simulink model "Simulacion_stepper"  (R2025b)
settings: Solver=ode4  StartTime=0.0  StopTime=Time_simulation  FixedStep=1/frecuency_simulation  RelTol=1e-3
InitFcn:
  | %%InitFcn();
StopFcn:
  | %%FinishFcn
model workspace (MAT data in the model file):
  Ts_stepper = 0.001
values from neighbouring files (symbols this model uses):
  B = motor_params.B_internal    [bode.m]    (also in current_observer.m = 0.0005; discretizacion.m = [ 1/L, 0; ekf_4_estados.m = params.B; obs_ctrl_back_emf_ext.m = [1/L 0)
  frecuency_simulation = 10e3    (= 10000)    [InitFcn.m]
  J = motor_params.J_internal    [bode.m]    (also in current_observer.m = 0.008; ekf_4_estados.m = params.J; obs_ctrl_back_emf_ext.m = 0.008; obs_y_contrl_back_emd.m = 0.008)
  Ke = 0.0055    [current_observer.m]    (also in ekf_4_estados.m = params.Ke; observer.m = Pvec(3); salient_motor.m = 0.0066)
  Ki_d = PI_dq_params.Ki_d_salient    [bode.m]
  Ki_q = PI_dq_params.Ki_q_salient    [bode.m]
  Ki_w = (wn_w^2)*J_var/Kt    [Barrido_B.m]    (also in Barrido_J.m; bode.m = PI_MTPA_params.Ki_w)
  Kp_d = PI_dq_params.Kp_d_salient    [bode.m]
  Kp_q = PI_dq_params.Kp_q_salient    [bode.m]
  Kp_w = (2*shi_w*wn_w*J_var)/Kt    [Barrido_B.m]    (also in Barrido_J.m; bode.m = PI_MTPA_params.Kp_w)
  Kt = Nr*Ke    (= 0.275)    [current_observer.m]    (also in ekf_4_estados.m = params.Kt; frecuencia_max.m = 0.33; observer.m = Pvec(4); salient_motor.m = 0.33)
  L = place(A', C', 10*eig(A)).'    [current_observer.m]    (also in desfase.m = lags(k); discretizacion.m = 0.01; frecuencia_max.m = 0.006; obs_ctrl_back_emf_ext.m = 0.006)
  P = motor_params.P    [bode.m]    (also in ekf_4_estados.m = P_pred; frecuencia_max.m = 50; salient_motor.m = 50)
  R = motor_params.R    [bode.m]    (also in current_observer.m = 3.4; discretizacion.m = 3.4; ekf_4_estados.m = params.R; frecuencia_max.m = 3.4)
  sample_time = 1/frecuency_simulation    (= 0.0001)    [InitFcn.m]
  Ts_current = 1/f_current    (= 0.0001)    [InitFcn.m]
  Ts_Wm = Ts_current*10    (= 0.001)    [InitFcn.m]
  Vdc = 24    [InitFcn.m]    (also in frecuencia_max.m = 12)
undefined symbols (not defined in the file or in its folder): DiscIntNeverNeededParam, EKF_params, motor_params, RI_base
libraries: simulink x8, mcbeeMathTransformLib x3, spspowerguiLib x1
(part 4 of 5)

== matlab function Simulacion_stepper/Triggered Subsystem2/MATLAB Function ==
  data: U input; x_out output; X input; Ts input; Ke input; Kt input; R input; J input; Ld input; Lq input; Nr input; B input; wh input; b0 input; b1 input; b2 input; a1 input; a2 input; HFI_flag input
function x_out = ekf_dq_5states_tightly_coupled( ...
    U, X, Ts, Ke, Kt, R, J, Ld, Lq, Nr, B, ...
    wh, b0, b1, b2, a1, a2, HFI_flag)

% =========================================================================
% EKF 5 ESTADOS TIGHTLY COUPLED CON HFI
%
% Estados:
%
%   x = [Id; Iq; Wm; theta_e; Tx]
%
% theta_e:
%   Ángulo eléctrico.
%
% Mediciones:
%
%   y_med  = [Ia; Ib; 0]
%   y_pred = [Ia_pred; Ib_pred; eps_norm]
%
% La tercera medición impone:
%
%   eps_norm -> 0
%
% IMPORTANTE:
%   Para que esta formulación sea físicamente coherente, eps_norm debe
%   representar aproximadamente un error angular eléctrico.
% =========================================================================

% Parámetros no utilizados actualmente:
% N_steps, Tdtm, beta0, beta1, beta2

Ts_eff = max(Ts, 1e-9);

% =========================================================================
% ESTADOS PERSISTENTES
% =========================================================================

persistent x_hat
persistent P
persistent Qk

persistent xa1 xa2 ya1 ya2
persistent xb1 xb2 yb1 yb2

persistent t_h
persistent eps_f

if isempty(x_hat)

    % Estado inicial
    x_hat = zeros(5,1);

    % Covarianza inicial
    P = diag([ ...
        1e-6, ...   % Id
        1e-6, ...   % Iq
        1e-6, ...   % Wm
        1e-9, ...   % theta_e
        1e-5]);     % Tx

    % Ruido del proceso
    Qk = diag([ ...
        1e-8, ...   % Id
        1e-8, ...   % Iq
        1e-8, ...   % Wm
        1e-12, ...   % theta_e
        1e-5]);     % Tx

    % Estados del BPF de Ia
    xa1 = 0;
    xa2 = 0;
    ya1 = 0;
    ya2 = 0;

    % Estados del BPF de Ib
    xb1 = 0;
    xb2 = 0;
    yb1 = 0;
    yb2 = 0;

    % Estados HFI
    t_h   = 0;
    eps_f = 0;

end

% =========================================================================
% 1. MEDICIONES Y ENTRADAS
% =========================================================================

Ia_raw = X(1);
Ib_raw = X(2);

Va = U(1);
Vb = U(2);

% =========================================================================
% 2. ESTADOS ACTUALES
% =========================================================================

Id = x_hat(1);
Iq = x_hat(2);
Wm = x_hat(3);

% El estado angular se conserva continuo internamente
theta_e_state = x_hat(4);

Tx = x_hat(5);

% Ángulo envuelto únicamente para trigonometría
theta_e = wrap_pi(theta_e_state);

c = cos(theta_e);
s = sin(theta_e);

% =========================================================================
% 3. TRANSFORMACIÓN DE TENSIONES AL MARCO dq
% =========================================================================

Vd =  Va*c + Vb*s;
Vq = -Va*s + Vb*c;

% =========================================================================
% 4. PREDICCIÓN DEL ESTADO
% =========================================================================

We = Nr*Wm;

dId = ( ...
      Vd ...
    - R*Id ...
    + We*Lq*Iq) / Ld;

dIq = ( ...
      Vq ...
    - R*Iq ...
    - We*Ld*Id ...
    - Ke*Wm) / Lq;

% Torque electromagnético
Te = Kt*Iq + Nr*(Lq-Ld)*Id*Iq;

% Tx representa la carga desconocida
dWm = (Te - B*Wm - Tx)/J;

% Alternativa si Tdtm es una carga conocida:
%
% dWm = (Te - B*Wm - Tdtm - Tx)/J;

x_pred = zeros(5,1);

x_pred(1) = Id + Ts_eff*dId;
x_pred(2) = Iq + Ts_eff*dIq;
x_pred(3) = Wm + Ts_eff*dWm;

% Ángulo eléctrico continuo
x_pred(4) = theta_e_state + Ts_eff*Nr*Wm;

% Torque desconocido como random walk
x_pred(5) = Tx;

% =========================================================================
% 5. JACOBIANA DE TRANSICIÓN
% =========================================================================

A = [ ...
    -R/Ld, ...
     Nr*Wm*Lq/Ld, ...
     Nr*Lq*Iq/Ld, ...
     Vq/Ld, ...
     0;

    -Nr*Wm*Ld/Lq, ...
    -R/Lq, ...
    -(Nr*Ld*Id + Ke)/Lq, ...
    -Vd/Lq, ...
     0;

     Nr*(Lq-Ld)*Iq/J, ...
     (Kt + Nr*(Lq-Ld)*Id)/J, ...
    -B/J, ...
     0, ...
    -1/J;

     0, ...
     0, ...
     Nr, ...
     0, ...
     0;

     0, ...
     0, ...
     0, ...
     0, ...
     0];

Phi = eye(5) + Ts_eff*A;

P_pred = Phi*P*Phi' + Qk;
P_pred = 0.5*(P_pred + P_pred');

% =========================================================================
% 6. FILTRO PASABANDA DE LAS CORRIENTES HFI
% =========================================================================

Iah = ...
      b0*Ia_raw ...
    + b1*xa1 ...
    + b2*xa2 ...
    - a1*ya1 ...
    - a2*ya2;

xa2 = xa1;
xa1 = Ia_raw;

ya2 = ya1;
ya1 = Iah;

Ibh = ...
      b0*Ib_raw ...
    + b1*xb1 ...
    + b2*xb2 ...
    - a1*yb1 ...
    - a2*yb2;

xb2 = xb1;
xb1 = Ib_raw;

yb2 = yb1;
yb1 = Ibh;

% =========================================================================
% 7. PROYECCIÓN HFI RESPECTO DEL ÁNGULO PREDICHO
% =========================================================================

theta_e_pred = wrap_pi(x_pred(4));

ch = cos(theta_e_pred);
sh = sin(theta_e_pred);

% Componente HFI sobre el eje q estimado
Iqh = -Iah*sh + Ibh*ch;

% =========================================================================
% 8. DEMODULACIÓN SÍNCRONA
% =========================================================================

if wh > 0

    t_h = t_h + Ts_eff;

    T_hfi = 2*pi/wh;

    if t_h >= T_hfi
        t_h = t_h - T_hfi*floor(t_h/T_hfi);
    end

    % Verificar signo y fase según la señal efectivamente inyectada
    eps_raw = -Iqh*cos(wh*t_h);

else

    t_h = 0;
    eps_raw = 0;

end

% =========================================================================
% 9. FILTRO PASABAJOS DEL ERROR HFI
% =========================================================================

f_lpf_hfi = 50;

tau_lpf   = 1/(2*pi*f_lpf_hfi);
alpha_lpf = Ts_eff/(Ts_eff + tau_lpf);

eps_f = eps_f + alpha_lpf*(eps_raw - eps_f);

% =========================================================================
% 10. NORMALIZACIÓN DEL ERROR HFI
% =========================================================================

DeltaL = Lq - Ld;
Lavg   = 0.5*(Ld + Lq);

if abs(DeltaL) < 1e-12 || Lavg <= 0

    eps_norm = 0;

else

    saliency = DeltaL/Lavg;

    % Formulación original:
    %
    % Se supone empíricamente que eps_norm aproxima un error angular.
    %
    % Atención: dividir por la saliencia no garantiza que el resultado
    % tenga unidades de radianes.
    % Formulación original:
    eps_norm = eps_f/abs(saliency);
    
    % NUEVO: Límite estricto de seguridad para evitar retroalimentación positiva
    max_eps = pi/4; % 45 grados eléctricos
    eps_norm = max(-max_eps, min(max_eps, eps_norm));

end

if ~HFI_flag
    eps_norm = 0;
end

% Protección numérica
if ~isfinite(eps_norm)
    eps_norm = 0;
end

% =========================================================================
% 11. PREDICCIÓN DE LAS MEDICIONES DE CORRIENTE
% =========================================================================

Id_p = x_pred(1);
Iq_p = x_pred(2);

cp = cos(theta_e_pred);
sp = sin(theta_e_pred);

Ia_pred = Id_p*cp - Iq_p*sp;
Ib_pred = Id_p*sp + Iq_p*cp;

% =========================================================================
% 12. VECTOR DE MEDICIÓN DE TRES COMPONENTES
% =========================================================================
%
% La tercera medición impone que el error HFI sea cero.
% =========================================================================

y_med = [ ...
    Ia_raw;
    Ib_raw;
    0];

y_pred = [ ...
    Ia_pred;
    Ib_pred;
    eps_norm];

innov = y_med - y_pred;

% Equivalente:
%
% innov(1) = Ia_raw - Ia_pred
% innov(2) = Ib_raw - Ib_pred
% innov(3) = -eps_norm

% =========================================================================
% 13. JACOBIANA DE MEDICIÓN
% =========================================================================

dIa_dtheta_e = -Id_p*sp - Iq_p*cp;
dIb_dtheta_e =  Id_p*cp - Iq_p*sp;

% Si:
%
% eps_norm ≈ theta_real - theta_estimado
%
% entonces:
%
% d(eps_norm)/d(theta_estimado) ≈ -1
dEps_dtheta_e = -1;

Ck = [ ...
    cp, -sp, 0, dIa_dtheta_e, 0;
    sp,  cp, 0, dIb_dtheta_e, 0;
    0,   0,  0, dEps_dtheta_e, 0];

% =========================================================================
% 14. COVARIANZA DE LAS TRES MEDICIONES
% =========================================================================

sigma_Ia = 0.1;
sigma_Ib = 0.1;

if HFI_flag

    sigma_HFI = 0.25;

else

    % El HFI queda prácticamente ignorado
    sigma_HFI = 1e6;

end

Rk = diag([ ...
    sigma_Ia^2, ...
    sigma_Ib^2, ...
    sigma_HFI^2]);

% =========================================================================
% 15. GANANCIA DE KALMAN
% =========================================================================

Sk = Ck*P_pred*Ck' + Rk;
Sk = 0.5*(Sk + Sk');

% Evitar inversión explícita
Lk = (P_pred*Ck')/Sk;

% =========================================================================
% 16. CORRECCIÓN TIGHTLY COUPLED
% =========================================================================

x_corr_ekf = x_pred + Lk*innov;

% No se envuelve internamente para mantener continuidad angular
% x_corr_ekf(4) permanece continuo.

% =========================================================================
% 17. ACTUALIZACIÓN DE COVARIANZA: FORMA DE JOSEPH
% =========================================================================

I5 = eye(5);

P = ...
    (I5 - Lk*Ck)*P_pred*(I5 - Lk*Ck)' ...
    + Lk*Rk*Lk';

P = 0.5*(P + P');

% =========================================================================
% 18. PROTECCIÓN NUMÉRICA
% =========================================================================

if any(~isfinite(x_corr_ekf)) || any(~isfinite(P(:)))

    x_corr_ekf = x_pred;
    P = P_pred;

end

% =========================================================================
% 19. ACTUALIZACIÓN DEL ESTADO
% =========================================================================

x_hat = x_corr_ekf;

% =========================================================================
% 20. SALIDA
% =========================================================================

x_out = x_hat;

% Solo la salida angular se envuelve
x_out(4) = wrap_pi(x_hat(4));

end

% =========================================================================
% FUNCIÓN AUXILIAR
% =========================================================================

function out = wrap_pi(in)

out = atan2(sin(in), cos(in));

end

== matlab function Simulacion_stepper/Triggered Subsystem2/MATLAB Function1 ==
  data: U input; x_corr output; X input; Ts input; Kt input; R input; J input; L input; Nr input; B input; Ke input
function x_corr = ekf_5var(U,X,Ts,Kt,R,J,L,Nr,B,Ke)
persistent x_hat P x_pred
%%  x_hat son los estados predichos
%%  x_corr es la salida corregida
%%  P_pre ó Sum_less es la covarianza predicha
%%  P ó sum_more es la covarianza
%%  Rk ó sum_v es la covarianza de incertidumbre del sensor




 %%Iniciamos calculando X_hat[k-1]
 if isempty(x_hat)
     x_hat = zeros(5,1);
     P = diag([1e-4 1e-4 1e-6 1e-10 1e-4]);
     x_corr = zeros(5,1);
     x_pred = zeros(5,1);


 end

Qk = diag([1e-4 1e-4 1e-4 1e-10 1e-6]);
Rk = diag([5e-4 5e-4]);   % ruido de medición

%%1A
%%Predicción
Ia = x_hat(1);
Ib = x_hat(2);
Wm = x_hat(3);
Th_m = x_hat(4);
Tx = x_hat(5);

Th_e = Nr*Th_m;
S = sin(Th_e);
C = cos(Th_e);

Va = U(1);
Vb = U(2);

dx = zeros(5,1);
dx(1) = (Va - R*Ia + Ke*Wm*S)/L;
dx(2) = (Vb - R*Ib - Ke*Wm*C)/L;
dx(3) = (Kt*(Ib*C-Ia*S) -Tx)/J;
dx(4) = Wm;
dx(5) = 0;
x_pred = x_hat + Ts*dx;
x_pred(4) = wrap_2pi(x_pred(4));

%%Calculamos el jacobiano
RL = R/L;
uno = Ke*S;
dos = Ke*C;

A = [-RL 0   (uno/L) (dos*Nr*Wm/L) 0;
 0  -RL   -dos/L    uno*Nr*Wm/L  0;
 -uno/J dos/J -1/J -Kt*Nr*(Ia*C+Ib*S)/J -1/J;
 0 0 1 0 0;
 0 0 0 0 0];

A_hat = eye(5) + Ts*A;
A_hat_T = transpose(A_hat);

%%1B COVARIANZA PREDICHA
P_pred = A_hat * P * A_hat_T + Qk; 


%%1C PREDECIMOS LA SALIDA DEL SISTEMA
Ck = [1 0 0 0 0;
      0 1 0 0 0];
Ck_T = transpose(Ck);
y_pred = Ck*x_pred;

%%2A calculamos la matriz Lk
%%Lk = P_pred *Ck_T * inv(Ck*P_pred*Ck_T + sum_v)
Sk = Ck*P_pred*Ck_T + Rk;
Lk = P_pred * Ck_T /Sk;

%%2B Actualizamos los estados estados corregidos en función de L


y_meas = [X(1);X(2)];

innov = y_meas - y_pred;
x_corr = x_pred + Lk*(innov);
x_corr(4) = wrap_2pi(x_corr(4));
%%actualizamos la covarianza y guardamos el estado
x_hat = x_corr;
Lk_T = transpose(Lk);
P = P_pred - Lk*Sk*Lk_T;
P_T = transpose(P);
P = 0.5 * (P + P_T);

== matlab function Simulacion_stepper/Triggered Subsystem2/MATLAB Function2 ==
  data: U input size=2; x_corr output; Y input size=2; Ts input; Kt input; R input; J input; L input; Nr input; B input
function x_corr = SPKF_4var(U,Y,Ts,Kt,R,J,L,Nr,B)
persistent x_hat P  alpham alphac Qk Rk h
%%  x_hat son los estados predichos
%%  x_corr es la salida corregida
%%  P_pre ó Sum_less es la covarianza predicha
%%  P ó sum_more es la covarianza
%%  Rk ó sum_v es la covarianza de incertidumbre del sensor


Nx = 4; %%Números de estados
Nw = 4; %% Incertidumbres de estado
Ny = 2; %% Incertidumbre de mediciones
Na = Nx+Nw+Ny;


%%Los métodos de sigma-point pueden diferir al utilizar las variables
%%alpha. Existen 2 métodos:

%% Método |    Sigma       |     alpha_m_0      | alpha_m_k         |           alpha_c_0               | alpha_c_k |
%% UKF    | sqrt(L+lambda) |  lambda/(L+Lambda) | 1/(2*(L+Lambda))  | alpha_m_0 + (1-alpha^2 + betha)   | alpha_m_k |
%% CDKF   |    h           |   (h^2 - L)/h^2    |  1/(2*h^2)        | alpha_m_0                         | alpha_m_k |
 %%Iniciamos calculando X_hat[k-1]
 if isempty(x_hat)
    
     %%Utilizamos el CDKF, con h = sqrt(Nxa); 
        x_hat = zeros(Nx,1);
        h =sqrt(Na);
        alpham = ones(2*Na+1,1) * (1/(2*h^2));
        alpham(1) = (h^2 - Na)/(h^2);   % peso del sigma central
        alphac = alpham;             
     %%Valores de covarianza
     P = diag([1e-2 1e-2 1e-6 1e-12 ]);
     Qk = diag([1e-2 1e-2 1e-8 1e-12 ]);
     Rk = [1e-4 0; 0 1e-4];
 end
    
     x_corr = zeros(Nx,1);
     x_pred = zeros(Nx,1);
     x_hat_a = zeros(Na,1);
     X_minus = zeros(Nx,2*Na+1);
     Y_minus = zeros(Ny,2*Na+1);
%%Ciclo de 2*Na+1
%%Aun que deberiamos hacer un ciclo for, en matlab se hace solo asi que no
%%es necesario

%% 1A-I Creamos el vector de estados extendidos
x_hat_a = [x_hat;zeros(Nw,1);zeros(Ny,1)]; 


%% 1A-II Conseguimos el factor de cholesky


%%Creamos la matriz de covarianza extendidas, el cual es de la forma
%%             [P   0    0]
%%     P_a =   [0   Qk   0]
%%             [0   0   Rk]

P_a = blkdiag(P,Qk,Rk);
Sa = chol(P_a,"lower");

%% 1A-III generamos los sigma points
%% Queda de la forma [x_hat_a, x_hat_a + h*S,x_hat_a - h*S] (Por eso es 2*Nxa+1 = N)
%% Al usar x_a x_a(:,ones(1,Na)) creamos una matriz de la forma [x_a,x_a...x_a], que es de tamaño (Na)x(2*Na+1)
%% Posteriormente, se le suma un vector de [0,+h*S,-h*S]
%% Cómo S es del tamaño (Nxa)x(Nxa), el total es de (2*Na+1 = N)
X =  x_hat_a(:,ones(1,2*Na+1)) + h*[zeros(Na,1), Sa, -Sa];

%% 1A-IV Calculamos las ecuaciones de estado
Va = U(1);
Vb = U(2);


for k=1:2*Na+1

  % --- separar estado, ruido de proceso y ruido de medición ---


xk = X(1:Nx,k);                     % [Ia; Ib; Wm; Th_m]
wk = X(Nx+1 : Nx+Nw,k);             % ruido de proceso (4x1)
vk = X(Nx+Nw+1 : end,k);            % ruido de medición (2x1)    

Ia = xk(1);
Ib = xk(2);
Wm = xk(3);
Th_m = xk(4);

Th_e = Nr*Th_m;
S = sin(Th_e);
C = cos(Th_e);


dx1 = (Va - R*Ia + Kt*Wm*S)/L;
dx2 = (Vb - R*Ib - Kt*Wm*C)/L;
dx3 = (Kt*(Ib*C-Ia*S)-B*Wm)/J;
dx4 = Wm;

%Calculamos el paso siguiente mediante euler
%% X_minus corresponde a la matriz que contiene todos los sigma-points distribuidos en los estados del sistema no-extendido (Nx)x(Na)
X_minus(1,k) = Ia + Ts*dx1+ wk(1);
X_minus(2,k) = Ib + Ts*dx2 + wk(2);
X_minus(3,k) = Wm + Ts*dx3 + wk(3);
X_minus(4,k) = Th_m + Ts*dx4 + wk(4);
%%X_minus(4,k) = wrap_2pi(X_minus(4,k));

Y_minus(1,k) = X_minus(1,k) + vk(1);
Y_minus(2,k) = X_minus(2,k) + vk(2);

end
%% 1B Reconstrucción de la media
%% Esta matriz contiene la media de todos los estados. (Nx)x(1)
x_pred = X_minus*alpham;
y_pred = Y_minus*alpham;
%%  Reconstrucción de la covarianza

%% Acá lo que hacemos es copiar la media N veces, para poder realizar la resta.
%%Pero realmente debería ser un for de [Xs(i,k)= X_minus(i,k) - x_pred(i)],
%%dónde K es cada variable de estado (Nx)
%% Xs es una matriz de desviación respecto a la media. Es necesario para construir la covarianza P
Xs = X_minus - x_pred(:,ones([1 2*Na+1])); 
Ys = Y_minus - y_pred(:,ones([1 2*Na+1]));

Xs_T = transpose(Xs);
Ys_T = transpose(Ys);
%%Calculamos la matriz de covarianza, pero hay que considerar que como
%%diag(alphac) es una matriz llena de diagonales, uno puede reducir la
%%cantidad de cómputo.
P_pred = Xs*diag(alphac)*Xs_T;
Pyy = Ys* diag(alphac)* Ys_T;
Pxy = Xs*diag(alphac)*Ys_T;
Lk = Pxy/Pyy;
Lk_T = transpose(Lk);
%% 2B Leemos la medición y actualizamos
x_corr = x_pred + Lk*(Y - y_pred);
x_corr(4) = wrap_2pi(x_corr(4));
%%Guardamos los valores de x_hat para mantenerlos
x_hat = x_corr; 
%% 2C Actualizamos la covarianza
P = P_pred - Lk*Pyy*Lk_T;
P_T = transpose(P);
P = 0.5 * (P + P_T);

== matlab function Simulacion_stepper/Triggered Subsystem2/MATLAB Function3 ==
  data: U input size=2; x_corr output; Y input size=2; Ts input; Kt input; R input; J input; L input; Nr input; B input
function x_corr = SPKF_5var(U,Y,Ts,Kt,R,J,L,Nr,B)
persistent x_hat P x_pred alpham alphac Qk Rk h
%%  x_hat son los estados predichos
%%  x_corr es la salida corregida
%%  P_pre ó Sum_less es la covarianza predicha
%%  P ó sum_more es la covarianza
%%  Rk ó sum_v es la covarianza de incertidumbre del sensor


Nx = 5; %%Números de estados
Nw = 5; %% Incertidumbres de estado
Ny = 2; %% Incertidumbre de mediciones
Na = Nx+Nw+Ny;


%%Los métodos de sigma-point pueden diferir al utilizar las variables
%%alpha. Existen 2 métodos:

%% Método |    Sigma       |     alpha_m_0      | alpha_m_k         |           alpha_c_0               | alpha_c_k |
%% UKF    | sqrt(L+lambda) |  lambda/(L+Lambda) | 1/(2*(L+Lambda))  | alpha_m_0 + (1-alpha^2 + betha)   | alpha_m_k |
%% CDKF   |    h           |   (h^2 - L)/h^2    |  1/(2*h^2)        | alpha_m_0                         | alpha_m_k |
 %%Iniciamos calculando X_hat[k-1]
 if isempty(x_hat)
    
     %%Utilizamos el CDKF, con h = sqrt(Nxa); 
        x_hat = zeros(Nx,1);
        h =sqrt(Na);
        alpham = ones(2*Na+1,1) * (1/(2*h^2));
        alpham(1) = (h^2 - Na)/(h^2);   % peso del sigma central
        alphac = alpham;             
     %%Valores de covarianza
     P = diag([1e-2 1e-2 1e-4 1e-8 1e-12]);
     Qk = diag([1e-2 1e-2 1e-6 1e-8 1e-12]);
     Rk = [1e-4 0; 0 1e-4];
 end
    
     x_corr = zeros(Nx,1);
     x_pred = zeros(Nx,1);
     x_hat_a = zeros(Na,1);
     X_minus = zeros(Nx,2*Na+1);
     Y_minus = zeros(Ny,2*Na+1);
%%Ciclo de 2*Na+1
%%Aun que deberiamos hacer un ciclo for, en matlab se hace solo asi que no
%%es necesario

%% 1A-I Creamos el vector de estados extendidos
x_hat_a = [x_hat;zeros(Nw,1);zeros(Ny,1)]; 


%% 1A-II Conseguimos el factor de cholesky


%%Creamos la matriz de covarianza extendidas, el cual es de la forma
%%             [P   0    0]
%%     P_a =   [0   Qk   0]
%%             [0   0   Rk]

P_a = blkdiag(P,Qk,Rk);
Sa = chol(P_a,"lower");

%% 1A-III generamos los sigma points
%% Queda de la forma [x_hat_a, x_hat_a + h*S,x_hat_a - h*S] (Por eso es 2*Nxa+1 = N)
%% Al usar x_a x_a(:,ones(1,Na)) creamos una matriz de la forma [x_a,x_a...x_a], que es de tamaño (Na)x(2*Na+1)
%% Posteriormente, se le suma un vector de [0,+h*S,-h*S]
%% Cómo S es del tamaño (Nxa)x(Nxa), el total es de (2*Na+1 = N)
X =  x_hat_a(:,ones(1,2*Na+1)) + h*[zeros(Na,1), Sa, -Sa];

%% 1A-IV Calculamos las ecuaciones de estado
Va = U(1);
Vb = U(2);


for k=1:2*Na+1

  % --- separar estado, ruido de proceso y ruido de medición ---


xk = X(1:Nx,k);                     % [Ia; Ib; Wm; Th_m]
wk = X(Nx+1 : Nx+Nw,k);             % ruido de proceso (4x1)
vk = X(Nx+Nw+1 : end,k);            % ruido de medición (2x1)    

Ia = xk(1);
Ib = xk(2);
Wm = xk(3);
Th_m = xk(4);
Tx = xk(5);

Th_e = Nr*Th_m;
S = sin(Th_e);
C = cos(Th_e);


dx1 = (Va - R*Ia + Kt*Wm*S)/L;
dx2 = (Vb - R*Ib - Kt*Wm*C)/L;
dx3 = (Kt*(Ib*C-Ia*S)-B*Wm - Tx)/J;
dx4 = Wm;
dTx = 0;

%Calculamos el paso siguiente mediante euler
%% X_minus corresponde a la matriz que contiene todos los sigma-points distribuidos en los estados del sistema no-extendido (Nx)x(Na)
X_minus(1,k) = Ia + Ts*dx1+ wk(1);
X_minus(2,k) = Ib + Ts*dx2 + wk(2);
X_minus(3,k) = Wm + Ts*dx3 + wk(3);
X_minus(4,k) = Th_m + Ts*dx4 + wk(4);
X_minus(4,k) = wrap_2pi(X_minus(4,k));
X_minus(5,k) = Tx + Ts*dTx + wk(5);

Y_minus(1,k) = X_minus(1,k) + vk(1);
Y_minus(2,k) = X_minus(2,k) + vk(2);

end
%% 1B Reconstrucción de la media
%% Esta matriz contiene la media de todos los estados. (Nx)x(1)
x_pred = X_minus*alpham;
y_pred = Y_minus*alpham;
%%  Reconstrucción de la covarianza

%% Acá lo que hacemos es copiar la media N veces, para poder realizar la resta.
%%Pero realmente debería ser un for de [Xs(i,k)= X_minus(i,k) - x_pred(i)],
%%dónde K es cada variable de estado (Nx)
%% Xs es una matriz de desviación respecto a la media. Es necesario para construir la covarianza P
Xs = X_minus - x_pred(:,ones([1 2*Na+1])); 
Ys = Y_minus - y_pred(:,ones([1 2*Na+1]));

Xs_T = transpose(Xs);
Ys_T = transpose(Ys);
%%Calculamos la matriz de covarianza, pero hay que considerar que como
%%diag(alphac) es una matriz llena de diagonales, uno puede reducir la
%%cantidad de cómputo.
P_pred = Xs*diag(alphac)*Xs_T;
Pyy = Ys* diag(alphac)* Ys_T;
Pxy = Xs*diag(alphac)*Ys_T;
Lk = Pxy/Pyy;
Lk_T = transpose(Lk);
%% 2B Leemos la medición y actualizamos
x_corr = x_pred + Lk*(Y - y_pred);
x_corr(4) = wrap_2pi(x_corr(4));
%%Guardamos los valores de x_hat para mantenerlos
x_hat = x_corr; 
%% 2C Actualizamos la covarianza
P = P_pred - Lk*Pyy*Lk_T;
P_T = transpose(P);
P = 0.5 * (P + P_T);

== matlab function Simulacion_stepper/Triggered Subsystem2/MATLAB Function4 ==
  data: U input; x_out output; X input; Ts input; Ke input; Kt input; R input; J input; Ld input; Lq input; Nr input; N_steps input; B input; d_hat output; Tdtm input; beta0 input; beta1 input; beta2 input; wh input; b0 input; b1 input; b2 input; a1 input; a2 input
function [x_out, d_hat] = ekf_dq_4states_final(U, X, Ts, Ke, Kt, R, J, Ld, Lq, Nr, N_steps, B, Tdtm, beta0, beta1, beta2, wh, b0, b1, b2, a1, a2)
% =========================================================================
% EKF + HFI EXTERNO TIPO PLL (CORREGIDO)
% =========================================================================
persistent x_hat P
persistent d_do theta_do omega_do
persistent xa1 xa2 ya1 ya2
persistent xb1 xb2 yb1 yb2
persistent t_h eps_f
persistent theta_hfi_e

if isempty(x_hat)
    x_hat = zeros(4,1);
    P = diag([1e-4, 1e-4, 1e-2, 1e-6]);
    d_do = 0;
    theta_do = 0;
    omega_do = 0;
    xa1 = 0; xa2 = 0; ya1 = 0; ya2 = 0;
    xb1 = 0; xb2 = 0; yb1 = 0; yb2 = 0;
    t_h = 0; eps_f = 0; theta_hfi_e = 0;
end

% 1. Corrientes medidas
Ia_raw = X(1); Ib_raw = X(2);

% 2. Ángulo eléctrico interno EKF
theta_e_ekf = wrap_pi(x_hat(4)*Nr);
c = cos(theta_e_ekf); s = sin(theta_e_ekf);

% 3. Transformación de Park
Id_m =  Ia_raw*c + Ib_raw*s;
Iq_m = -Ia_raw*s + Ib_raw*c;
Vd_m =  U(1)*c + U(2)*s;
Vq_m = -U(1)*s + U(2)*c;

% 4. EKF - Predicción (Modelo fundamental)
Id = x_hat(1); Iq = x_hat(2); Wm = x_hat(3);
dId = (Vd_m - R*Id + Nr*Wm*Lq*Iq)/Ld;
dIq = (Vq_m - R*Iq - Nr*Wm*Ld*Id - Ke*Wm)/Lq;

% Torque considerando saliencia real (Lq > Ld)
Te = Kt*Iq + Nr*(Ld - Lq)*Id*Iq;
dWm = (Te - B*Wm)/J; 
dTh = Wm;

x_pred = x_hat + Ts*[dId; dIq; dWm; dTh];
x_pred(4) = wrap_pi(x_pred(4));

% 5. Jacobiano continuo -> discreto
A = [ -R/Ld,                  Nr*Wm*Lq/Ld,             Nr*Lq*Iq/Ld,              0;
      -Nr*Wm*Ld/Lq,           -R/Lq,                  -(Nr*Ld*Id + Ke)/Lq,       0;
      Nr*(Ld-Lq)*Iq/J,        (Kt + Nr*(Ld-Lq)*Id)/J,  -B/J,                     0;
      0,                      0,                       1,                        0];
Phi = eye(4) + A*Ts;
Qk = diag([1e-6, 1e-6, 1e-4, 1e-9]);
P_pred = Phi*P*Phi' + Qk;

% 6. EKF - Corrección
Ck = [1 0 0 0; 0 1 0 0];
Rk = diag([1e-2, 1e-2]);
innov = [Id_m; Iq_m] - [x_pred(1); x_pred(2)];
Sk = Ck*P_pred*Ck' + Rk;
Lk = (P_pred*Ck')/Sk;

x_corr_ekf = x_pred + Lk*innov;
x_corr_ekf(4) = wrap_pi(x_corr_ekf(4));
P = (eye(4) - Lk*Ck)*P_pred;
P = 0.5*(P + P');

% 7. BPF para señales HFI
Iah = b0*Ia_raw + b1*xa1 + b2*xa2 - a1*ya1 - a2*ya2;
xa2 = xa1; xa1 = Ia_raw; ya2 = ya1; ya1 = Iah;

Ibh = b0*Ib_raw + b1*xb1 + b2*xb2 - a1*yb1 - a2*yb2;
xb2 = xb1; xb1 = Ib_raw; yb2 = yb1; yb1 = Ibh;

% 8. Park HFI con ángulo corregido
theta_e_ekf_corr = wrap_pi(x_corr_ekf(4)*Nr);
ch = cos(theta_e_ekf_corr); sh = sin(theta_e_ekf_corr);
Iqh = -Iah*sh + Ibh*ch;

% 9. Demodulación síncrona
t_h = t_h + Ts;
eps_raw = Iqh*sin(wh*t_h);

% 10. LPF HFI
f_lpf_hfi = 50; 
alpha_lpf = Ts/(Ts + 1/(2*pi*f_lpf_hfi));
eps_f = eps_f + alpha_lpf*(eps_raw - eps_f);

% 11. PLL HFI - Ajuste de signo por Saliencia Inversa
DeltaL = Lq - Ld; 
Lavg = 0.5*(Ld + Lq);
if abs(DeltaL) < 1e-12
    eps_norm = 0;
else
    saliency = DeltaL/Lavg;
    eps_norm = eps_f / abs(saliency);
end

K_hfi_pll = 1e-4; 
% NOTA: Signo MENOS para que el lazo busque estabilidad en el eje d (inductancia mínima)
theta_hfi_e = wrap_pi(theta_e_ekf_corr - K_hfi_pll*eps_norm); 

% 12. Compensación de Retraso de Fase (Delay Filtros)
theta_delay = 0.0; 
theta_hfi_e = wrap_pi(theta_hfi_e + theta_delay);

% 13. Transición Híbrida Inteligente EKF -> HFI
W_hfi_on  = 20; 
W_hfi_off = 30; 
if abs(x_corr_ekf(3)) <= W_hfi_on
    use_hfi = true;
elseif abs(x_corr_ekf(3)) >= W_hfi_off
    use_hfi = false;
else
    use_hfi = true;
end

theta_e_used = theta_e_ekf_corr;
if use_hfi
    theta_e_used = theta_hfi_e;
end
theta_m_used = wrap_pi(theta_e_used/Nr);

% =========================================================================
% 14. DISTURBANCE OBSERVER (Unificado en unidades mecánicas)
% =========================================================================
Id_c = x_corr_ekf(1); Iq_c = x_corr_ekf(2); theta_m_c = x_corr_ekf(4);

% El error se calcula en posición mecánica para mantener consistencia con J
e0_m = wrap_pi(theta_m_c - theta_do); 
Te_obs = Kt*Iq_c + Nr*(Ld - Lq)*Id_c*Iq_c;

% Integración del observador mecánico puramente lineal
theta_do = wrap_pi(theta_do + Ts*(omega_do + beta0*e0_m));
omega_do = omega_do + Ts*((Te_obs - d_do - B*omega_do)/J + beta1*e0_m);
d_do = d_do - Ts*beta2*e0_m;

% La salida d_hat estima la fricción y TODO el cogging de golpe
d_hat = d_do; 

% 15. Asignación de Estados Finales
x_out = x_corr_ekf;
x_out(4) = theta_m_used; % Inyección del ángulo híbrido para el control exterior
x_hat = x_corr_ekf;      % Mantener el core del EKF guiado por el modelo fundamental
end

function out = wrap_pi(in)
    out = atan2(sin(in), cos(in));
end

== matlab function Simulacion_stepper/Triggered Subsystem2/MATLAB Function5 ==
  data: U input size=[2 1]; x_out output size=[5 1]; X input size=[2 1]; EKF_params parameter; theta_m_hat output; theta_e_out output
function [x_out,theta_m_hat,theta_e_out]  = ...
    fcn(U, X, EKF_params)

[x_out,theta_m_hat,theta_e_out] = ekf_5_estados( ...
    U, X, EKF_params);
end

== matlab function Simulacion_stepper/MATLAB Function9 ==
  data: u input; y output
function y = fcn(u)

y = wrap_2pi(u);

== matlab function Simulacion_stepper/MATLAB Function10 ==
  data: u input; y output
function y = fcn(u)

y = wrap_2pi(u);

== matlab function Simulacion_stepper/MATLAB Function12 ==
  data: u input; y output
function y = fcn(u)

y = wrap_2pi(u);

== matlab function Simulacion_stepper/MATLAB Function14 ==
  data: u input; y output
function y = fcn(u)

y = wrap_2pi(u);

== matlab function Simulacion_stepper/Motor 2  Speed PR/MATLAB Function ==
  data: Wm_ref input; Wm input; Ts input; Kp_w input; Ki_w input; Kd_w input; Tf_w input; Tl_tdm input; B input; Imax input; RI_enable input; a_ri input; b_ri input; c_ri input; d_ri input; Kr_norm input; Ld input; Iq_ref output; Id_ref output; Iq_cogging output; Iq_PI output; Lq input; Ke input; P input; error_Wm output
function [Iq_ref, Id_ref, Iq_cogging, Iq_PI, error_Wm] = PI_speed_RI_MTPA( ...
        Wm_ref, Wm, Ts, ...
        Kp_w, Ki_w, Kd_w, Tf_w, ...
        Tl_tdm, B, ...
        Imax, ...
        RI_enable, a_ri, b_ri, c_ri, d_ri, Kr_norm, ...
        Ld, Lq, Ke, P)

% =========================================================================
% CONTROL DE VELOCIDAD Wm
%
% Incluye:
% - PI de velocidad.
% - Derivada opcional filtrada sobre la velocidad medida.
% - Compensación feedforward de carga/fricción.
% - Resonador opcional para cogging.
% - MTPA continuo.
% - Saturación vectorial de corriente.
% - Anti-windup del integrador de velocidad.
%
% Para usar solo PI:
%     Kd_w = 0;
%     RI_enable = 0;
% =========================================================================

% =========================================================================
% Estados persistentes
% =========================================================================
persistent int_w
persistent Wm_prev dWm_filt_prev
persistent y1_ri y2_ri
persistent e1_ri e2_ri

if isempty(int_w)

    int_w          = 0;

    Wm_prev        = 0;
    dWm_filt_prev  = 0;

    y1_ri          = 0;
    y2_ri          = 0;
    e1_ri          = 0;
    e2_ri          = 0;

end

% Protección numérica
Ts_eff   = max(Ts, 1e-9);
Imax_eff = max(abs(Imax), 1e-6);

% Constante de torque de reluctancia
Krel = P * (Lq - Ld);

% =========================================================================
% 1. Error de velocidad
% =========================================================================
error_Wm = Wm_ref - Wm;

% =========================================================================
% 2. Derivada filtrada sobre la velocidad medida
%
% Se usa derivada de Wm, no de error, para evitar golpes derivativos
% cuando cambia Wm_ref.
% =========================================================================
dWm_raw = (Wm - Wm_prev) / Ts_eff;

if Tf_w > 0
    alpha_d = Ts_eff / (Tf_w + Ts_eff);
    dWm_filt = dWm_filt_prev + alpha_d * (dWm_raw - dWm_filt_prev);
else
    dWm_filt = dWm_raw;
end

% Acción derivativa amortiguadora
D_w = -Kd_w * dWm_filt;

% =========================================================================
% 3. Feedforward de torque de carga y fricción
% =========================================================================
T_ff = Tl_tdm + B * Wm_ref;

if abs(Ke) > 1e-9
    Iq_ff = T_ff / Ke;
else
    Iq_ff = 0;
end

% =========================================================================
% 4. Resonador para compensación de ripple/cogging
% =========================================================================
if RI_enable == 1

    Iq_RI_new = ...
          c_ri * y1_ri ...
        - d_ri * y2_ri ...
        + Kr_norm * (error_Wm - a_ri * e1_ri + b_ri * e2_ri);

else
    Iq_RI_new = 0;
end

% =========================================================================
% 5. Integrador candidato
% =========================================================================
int_w_candidate = int_w + Ki_w * Ts_eff * error_Wm;

% =========================================================================
% 6. Cálculo PI/PID, MTPA y límite de corriente
%
% Se hacen hasta dos pasadas:
% - Primera: prueba integrando.
% - Segunda: si saturó y el integrador empeora la saturación,
%   se rechaza esa integración.
% =========================================================================
for pass = 1:2

    % Salida del controlador de velocidad
    Iq_PI = Kp_w * error_Wm + int_w_candidate + D_w;

    % Corriente q total solicitada
    Iq_ref_raw = Iq_ff + Iq_PI + Iq_RI_new;

    % =====================================================================
    % MTPA continuo
    %
    % Id_ref tiende suavemente a cero cuando Iq_ref_raw tiende a cero.
    % No existe umbral que fuerce saltos Id_ref = 0.
    % =====================================================================
    if abs(Krel) > 1e-9 && abs(Ke) > 1e-9

        A_mtpa = Ke / (2 * Krel);

        if abs(A_mtpa) > 1e-12

            % Forma numéricamente estable de:
            % Id = A - sign(A)*sqrt(A^2 + Iq^2)
            Id_ref_raw = -sign(A_mtpa) * (Iq_ref_raw^2) / ...
                (abs(A_mtpa) + sqrt(A_mtpa^2 + Iq_ref_raw^2));

        else
            Id_ref_raw = 0;
        end

    else
        Id_ref_raw = 0;
    end

    % =====================================================================
    % Saturación vectorial de corriente
    % =====================================================================
    Is_mag = sqrt(Id_ref_raw^2 + Iq_ref_raw^2);

    if Is_mag > Imax_eff

        ratio  = Imax_eff / Is_mag;

        Id_ref = Id_ref_raw * ratio;
        Iq_ref = Iq_ref_raw * ratio;

        sat = true;

    else

        Id_ref = Id_ref_raw;
        Iq_ref = Iq_ref_raw;

        sat = false;
    end

    % =====================================================================
    % Anti-windup condicional
    %
    % Si la salida está saturada y el error pide aumentar todavía más
    % la corriente saturada, no se integra.
    % Si el error ayuda a salir de saturación, sí se permite integrar.
    % =====================================================================
    integrator_worsens_sat = (Iq_ref_raw * error_Wm) >= 0;

    if pass == 1 && sat && integrator_worsens_sat

        % Rechaza la nueva integración y recalcula la salida.
        int_w_candidate = int_w;

    else
        break;
    end

end

% Guarda el integrador final
int_w = int_w_candidate;

% =========================================================================
% 7. Actualización de memorias
%
% Estas memorias se actualizan siempre, incluso durante saturación.
% =========================================================================
Wm_prev       = Wm;
dWm_filt_prev = dWm_filt;

if RI_enable == 1

    y2_ri = y1_ri;
    y1_ri = Iq_RI_new;

    e2_ri = e1_ri;
    e1_ri = error_Wm;

else

    % Evita que el resonador conserve memoria al desactivarlo.
    y1_ri = 0;
    y2_ri = 0;
    e1_ri = 0;
    e2_ri = 0;

end

% =========================================================================
% 8. Salidas de monitoreo
% =========================================================================
Iq_cogging = Iq_RI_new;

end

== matlab function Simulacion_stepper/Motor 2 PI Speed MTPA/MATLAB Function1 ==
  data: Wm_ref input size=1; T_ref output; Wm input size=1; tl_tdm input; T_PI output; error_Wm output; Wm_filt output; PI_MTPA_params parameter
function [T_ref, T_PI, error_Wm, Wm_filt] = ...
    fcn(Wm_ref, Wm, tl_tdm, PI_MTPA_params)

[T_ref, T_PI, error_Wm, Wm_filt] = ...
    PI_speed( ...
        Wm_ref, ...
        Wm, ...
        tl_tdm, ...
        PI_MTPA_params);

end

== matlab function Simulacion_stepper/Triggered Subsystem1/MATLAB Function4 ==
  data: U input; x_out output; X input; Ts input; Ke input; Kt input; R input; J input; Ld input; Lq input; Nr input; N_steps input; B input; d_hat output; Tdtm input; beta0 input; beta1 input; beta2 input; wh input; b0 input; b1 input; b2 input; a1 input; a2 input
function [x_out, d_hat] = ekf_dq_4states_final(U, X, Ts, Ke, Kt, R, J, Ld, Lq, Nr, N_steps, B, Tdtm, beta0, beta1, beta2, wh, b0, b1, b2, a1, a2)
% =========================================================================
% EKF + HFI EXTERNO TIPO PLL (CORREGIDO)
% =========================================================================
persistent x_hat P
persistent d_do theta_do omega_do
persistent xa1 xa2 ya1 ya2
persistent xb1 xb2 yb1 yb2
persistent t_h eps_f
persistent theta_hfi_e

if isempty(x_hat)
    x_hat = zeros(4,1);
    P = diag([1e-4, 1e-4, 1e-2, 1e-6]);
    d_do = 0;
    theta_do = 0;
    omega_do = 0;
    xa1 = 0; xa2 = 0; ya1 = 0; ya2 = 0;
    xb1 = 0; xb2 = 0; yb1 = 0; yb2 = 0;
    t_h = 0; eps_f = 0; theta_hfi_e = 0;
end

% 1. Corrientes medidas
Ia_raw = X(1); Ib_raw = X(2);

% 2. Ángulo eléctrico interno EKF
theta_e_ekf = wrap_pi(x_hat(4)*Nr);
c = cos(theta_e_ekf); s = sin(theta_e_ekf);

% 3. Transformación de Park
Id_m =  Ia_raw*c + Ib_raw*s;
Iq_m = -Ia_raw*s + Ib_raw*c;
Vd_m =  U(1)*c + U(2)*s;
Vq_m = -U(1)*s + U(2)*c;

% 4. EKF - Predicción (Modelo fundamental)
Id = x_hat(1); Iq = x_hat(2); Wm = x_hat(3);
dId = (Vd_m - R*Id + Nr*Wm*Lq*Iq)/Ld;
dIq = (Vq_m - R*Iq - Nr*Wm*Ld*Id - Ke*Wm)/Lq;

% Torque considerando saliencia real (Lq > Ld)
Te = Kt*Iq + Nr*(Ld - Lq)*Id*Iq;
dWm = (Te - B*Wm)/J; 
dTh = Wm;

x_pred = x_hat + Ts*[dId; dIq; dWm; dTh];
x_pred(4) = wrap_pi(x_pred(4));

% 5. Jacobiano continuo -> discreto
A = [ -R/Ld,                  Nr*Wm*Lq/Ld,             Nr*Lq*Iq/Ld,              0;
      -Nr*Wm*Ld/Lq,           -R/Lq,                  -(Nr*Ld*Id + Ke)/Lq,       0;
      Nr*(Ld-Lq)*Iq/J,        (Kt + Nr*(Ld-Lq)*Id)/J,  -B/J,                     0;
      0,                      0,                       1,                        0];
Phi = eye(4) + A*Ts;
Qk = diag([1e-6, 1e-6, 1e-4, 1e-9]);
P_pred = Phi*P*Phi' + Qk;

% 6. EKF - Corrección
Ck = [1 0 0 0; 0 1 0 0];
Rk = diag([1e-2, 1e-2]);
innov = [Id_m; Iq_m] - [x_pred(1); x_pred(2)];
Sk = Ck*P_pred*Ck' + Rk;
Lk = (P_pred*Ck')/Sk;

x_corr_ekf = x_pred + Lk*innov;
x_corr_ekf(4) = wrap_pi(x_corr_ekf(4));
P = (eye(4) - Lk*Ck)*P_pred;
P = 0.5*(P + P');

% 7. BPF para señales HFI
Iah = b0*Ia_raw + b1*xa1 + b2*xa2 - a1*ya1 - a2*ya2;
xa2 = xa1; xa1 = Ia_raw; ya2 = ya1; ya1 = Iah;

Ibh = b0*Ib_raw + b1*xb1 + b2*xb2 - a1*yb1 - a2*yb2;
xb2 = xb1; xb1 = Ib_raw; yb2 = yb1; yb1 = Ibh;

% 8. Park HFI con ángulo corregido
theta_e_ekf_corr = wrap_pi(x_corr_ekf(4)*Nr);
ch = cos(theta_e_ekf_corr); sh = sin(theta_e_ekf_corr);
Iqh = -Iah*sh + Ibh*ch;

% 9. Demodulación síncrona
t_h = t_h + Ts;
eps_raw = Iqh*sin(wh*t_h);

% 10. LPF HFI
f_lpf_hfi = 50; 
alpha_lpf = Ts/(Ts + 1/(2*pi*f_lpf_hfi));
eps_f = eps_f + alpha_lpf*(eps_raw - eps_f);

% 11. PLL HFI - Ajuste de signo por Saliencia Inversa
DeltaL = Lq - Ld; 
Lavg = 0.5*(Ld + Lq);
if abs(DeltaL) < 1e-12
    eps_norm = 0;
else
    saliency = DeltaL/Lavg;
    eps_norm = eps_f / abs(saliency);
end

K_hfi_pll = 1e-4; 
% NOTA: Signo MENOS para que el lazo busque estabilidad en el eje d (inductancia mínima)
theta_hfi_e = wrap_pi(theta_e_ekf_corr - K_hfi_pll*eps_norm); 

% 12. Compensación de Retraso de Fase (Delay Filtros)
theta_delay = 0.0; 
theta_hfi_e = wrap_pi(theta_hfi_e + theta_delay);

% 13. Transición Híbrida Inteligente EKF -> HFI
W_hfi_on  = 20; 
W_hfi_off = 30; 
if abs(x_corr_ekf(3)) <= W_hfi_on
    use_hfi = true;
elseif abs(x_corr_ekf(3)) >= W_hfi_off
    use_hfi = false;
else
    use_hfi = true;
end

theta_e_used = theta_e_ekf_corr;
if use_hfi
    theta_e_used = theta_hfi_e;
end
theta_m_used = wrap_pi(theta_e_used/Nr);

% =========================================================================
% 14. DISTURBANCE OBSERVER (Unificado en unidades mecánicas)
% =========================================================================
Id_c = x_corr_ekf(1); Iq_c = x_corr_ekf(2); theta_m_c = x_corr_ekf(4);

% El error se calcula en posición mecánica para mantener consistencia con J
e0_m = wrap_pi(theta_m_c - theta_do); 
Te_obs = Kt*Iq_c + Nr*(Ld - Lq)*Id_c*Iq_c;

% Integración del observador mecánico puramente lineal
theta_do = wrap_pi(theta_do + Ts*(omega_do + beta0*e0_m));
omega_do = omega_do + Ts*((Te_obs - d_do - B*omega_do)/J + beta1*e0_m);
d_do = d_do - Ts*beta2*e0_m;

% La salida d_hat estima la fricción y TODO el cogging de golpe
d_hat = d_do; 

% 15. Asignación de Estados Finales
x_out = x_corr_ekf;
x_out(4) = theta_m_used; % Inyección del ángulo híbrido para el control exterior
x_hat = x_corr_ekf;      % Mantener el core del EKF guiado por el modelo fundamental
end

function out = wrap_pi(in)
    out = atan2(sin(in), cos(in));
end

== matlab function Simulacion_stepper/Motor 2 PI dq/MATLAB Function1 ==
  data: Wm input; Vd output; X input; Theta_e input; T_ref input; comp_res input; Vq output; Id_out output; Iq_out output; Valpha output; Vbetha output; Vd_hfi output; Vq_hfi output; error_d output; error_q output; PI_dq_params2 parameter; Id_ref_out output; Iq_ref_out output; T_ref_real output
function [Vd, Vq, Id_out, Iq_out, ...
          Valpha, Vbetha, Vd_hfi, Vq_hfi, ...
          error_d, error_q, ...
          Id_ref_out, Iq_ref_out, T_ref_real] = ...
    fcn(Wm, X, Theta_e, T_ref,comp_res, PI_dq_params2)

[Vd, Vq, Id_out, Iq_out, ...
          Valpha, Vbetha, Vd_hfi, Vq_hfi, ...
          error_d, error_q, ...
          Id_ref_out, Iq_ref_out, T_ref_real] = ...
    PI_dq( ...
        Wm, ...
        X, ...
        Theta_e, ...
        T_ref,...
        comp_res,...
        PI_dq_params2);

end

== matlab function Simulacion_stepper/Triggered Subsystem1/MATLAB Function5 ==
  data: U input size=[2 1]; x_out output size=[5 1]; X input size=[2 1]; EKF_params parameter; theta_m_hat output; theta_e_out output
function [x_out,theta_m_hat,theta_e_out]  = ...
    fcn(U, X, EKF_params)

[x_out,theta_m_hat,theta_e_out] = ekf_5_estados( ...
    U, X, EKF_params);
end

== matlab function Simulacion_stepper/MATLAB Function1 ==
  data: u input; y output
function y = fcn(u)

y = wrap_2pi(u);

== matlab function Simulacion_stepper/Motor 2  Speed PR/MATLAB Function1 ==
  data: Wm_ref input size=1; Vq_res output; Wm input size=1; error_res output; RI_params_M2 parameter; V_inphase output; V_quadrature output
function [Vq_res, error_res, V_inphase, V_quadrature] = ...
    fcn(Wm_ref, Wm, RI_params_M2)

[Vq_res, error_res, V_inphase, V_quadrature] = ...
    resonant_speed( ...
        Wm_ref, Wm, RI_params_M2);

end

== matlab function Simulacion_stepper/MATLAB Function5 ==
  data: u input; y output
function y = fcn(u)

y = wrap_2pi(u);

== matlab function Simulacion_stepper/MATLAB Function3 ==
  data: u input; y output
function y = fcn(u)

y = wrap_2pi(u);
